simulink library "lib_TCML"  (R2015a)
settings: Solver=ode45  StartTime=0.0  StopTime=10.0  RelTol=1e-3
libraries: simulink x5
(part 3 of 7)

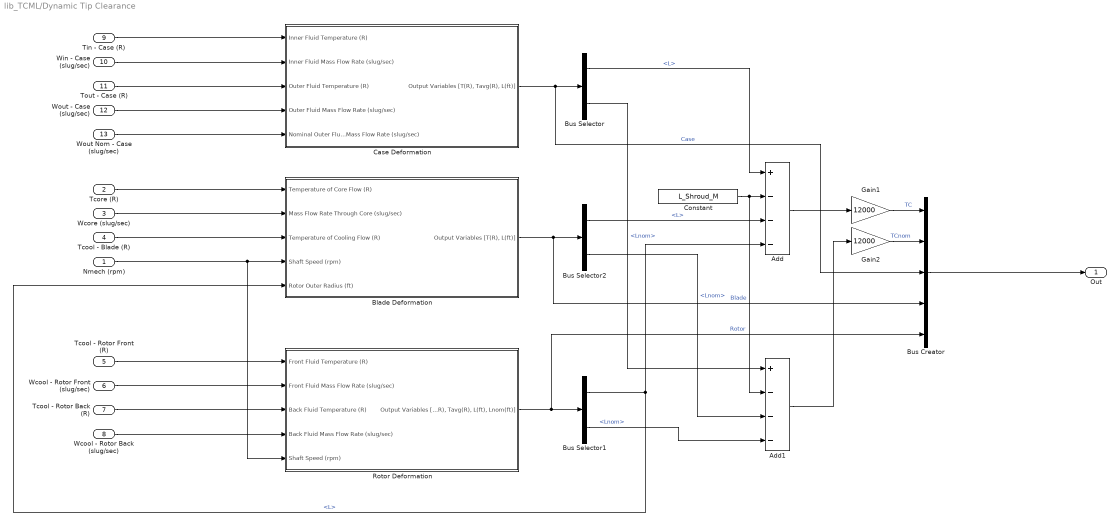
== system lib_TCML/Dynamic Tip Clearance ==
  Nmech (rpm) : Inport
  Tcore (R) : Inport  Port=2
  Wcore (slug/sec) : Inport  Port=3
  Tcool - Blade (R) : Inport  Port=4
  Tcool - Rotor Front (R) : Inport  Port=5
  Wcool - Rotor Front (slug/sec) : Inport  Port=6
  Tcool - Rotor Back (R) : Inport  Port=7
  Wcool - Rotor Back (slug/sec) : Inport  Port=8
  Tin - Case (R) : Inport  Port=9
  Win - Case (slug/sec) : Inport  Port=10
  Tout - Case (R) : Inport  Port=11
  Wout - Case (slug/sec) : Inport  Port=12
  Wout Nom - Case (slug/sec) : Inport  Port=13
  Add : Sum  Inputs=+---
  Add1 : Sum  Inputs=+---
  Blade Deformation : Subsystem
  Bus Creator : BusCreator  Inputs=5
  Bus Selector : BusSelector  OutputSignals=L,Lnom
  Bus Selector1 : BusSelector  OutputSignals=L,Lnom
  Bus Selector2 : BusSelector  OutputSignals=L,Lnom
  Case Deformation : Subsystem
  Constant : Constant  Value=L_Shroud_M
  Gain1 : Gain  Gain=12000
  Gain2 : Gain  Gain=12000
  Rotor Deformation : Subsystem
  Out : Outport
  wires:
  Add1/1 -> Gain2/1
  Bus Selector/2 -> Add1/1  "<Lnom>"
  Bus Selector2/2 -> Add1/3  "<Lnom>"
  Bus Selector1/2 -> Add1/4  "<Lnom>"
  Gain2/1 -> Bus Creator/2  "TCnom"
  Constant/1 -> Add/2, Add1/2
  Case Deformation/1("Output Variables [T(R), Tavg(R), L(ft)]") -> Bus Selector/1, Bus Creator/3  "Case"
  Wout - Case (slug/sec)/1 -> Case Deformation/4(Outer Fluid Mass Flow Rate (slug/sec))
  Tout - Case (R)/1 -> Case Deformation/3(Outer Fluid Temperature (R))
  Win - Case (slug/sec)/1 -> Case Deformation/2(Inner Fluid Mass Flow Rate (slug/sec))
  Tin - Case (R)/1 -> Case Deformation/1(Inner Fluid Temperature (R))
  Gain1/1 -> Bus Creator/1  "TC"
  Bus Selector/1 -> Add/1  "<L>"
  Bus Selector1/1 -> Add/4, Blade Deformation/5(Rotor Outer Radius (ft))  "<L>"
  Rotor Deformation/1("Output Variables [T(R), Tavg(R), L(ft), Lnom(ft)]") -> Bus Selector1/1, Bus Creator/5  "Rotor"
  Blade Deformation/1("Output Variables [T(R), L(ft)]") -> Bus Selector2/1, Bus Creator/4  "Blade"
  Bus Selector2/1 -> Add/3  "<L>"
  Add/1 -> Gain1/1
  Bus Creator/1 -> Out/1
  Tcore (R)/1 -> Blade Deformation/1(Temperature of Core Flow (R))
  Wcore (slug/sec)/1 -> Blade Deformation/2(Mass Flow Rate Through Core (slug/sec))
  Tcool - Blade (R)/1 -> Blade Deformation/3(Temperature of Cooling Flow (R))
  Nmech (rpm)/1 -> Blade Deformation/4(Shaft Speed (rpm)), Rotor Deformation/5(Shaft Speed (rpm))
  Tcool - Rotor Front (R)/1 -> Rotor Deformation/1(Front Fluid Temperature (R))
  Wcool - Rotor Front (slug/sec)/1 -> Rotor Deformation/2(Front Fluid Mass Flow Rate (slug/sec))
  Tcool - Rotor Back (R)/1 -> Rotor Deformation/3(Back Fluid Temperature (R))
  Wcool - Rotor Back (slug/sec)/1 -> Rotor Deformation/4(Back Fluid Mass Flow Rate (slug/sec))
  Wout Nom - Case (slug/sec)/1 -> Case Deformation/5(Nominal Outer Fluid Mass Flow Rate (slug/sec))

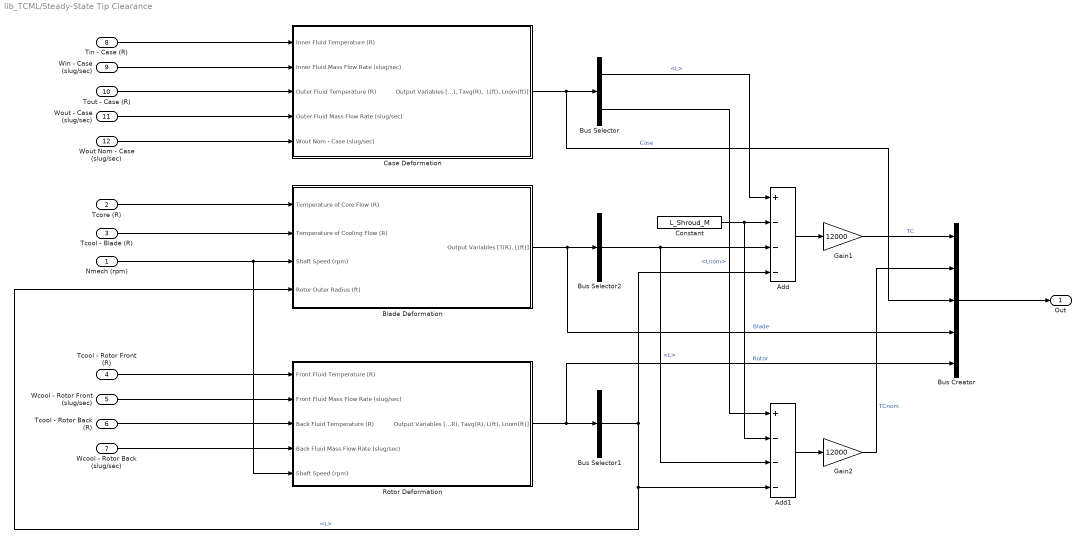
== system lib_TCML/Steady-State Tip Clearance ==
  Nmech (rpm) : Inport
  Tcore (R) : Inport  Port=2
  Tcool - Blade (R) : Inport  Port=3
  Tcool - Rotor Front (R) : Inport  Port=4
  Wcool - Rotor Front (slug/sec) : Inport  Port=5
  Tcool - Rotor Back (R) : Inport  Port=6
  Wcool - Rotor Back (slug/sec) : Inport  Port=7
  Tin - Case (R) : Inport  Port=8
  Win - Case (slug/sec) : Inport  Port=9
  Tout - Case (R) : Inport  Port=10
  Wout - Case (slug/sec) : Inport  Port=11
  Wout Nom - Case (slug/sec) : Inport  Port=12
  Add : Sum  Inputs=+---
  Add1 : Sum  Inputs=+---
  Blade Deformation : Subsystem
  Bus Creator : BusCreator  Inputs=5
  Bus Selector : BusSelector  OutputSignals=L,Lnom
  Bus Selector1 : BusSelector  OutputSignals=L
  Bus Selector2 : BusSelector  OutputSignals=L
  Case Deformation : Subsystem
  Constant : Constant  Value=L_Shroud_M
  Gain1 : Gain  Gain=12000
  Gain2 : Gain  Gain=12000
  Rotor Deformation : Subsystem
  Out : Outport
  wires:
  Tin - Case (R)/1 -> Case Deformation/1(Inner Fluid Temperature (R))
  Wcool - Rotor Back (slug/sec)/1 -> Rotor Deformation/4(Back Fluid Mass Flow Rate (slug/sec))
  Tcool - Rotor Back (R)/1 -> Rotor Deformation/3(Back Fluid Temperature (R))
  Wcool - Rotor Front (slug/sec)/1 -> Rotor Deformation/2(Front Fluid Mass Flow Rate (slug/sec))
  Tcool - Rotor Front (R)/1 -> Rotor Deformation/1(Front Fluid Temperature (R))
  Nmech (rpm)/1 -> Blade Deformation/3(Shaft Speed (rpm)), Rotor Deformation/5(Shaft Speed (rpm))
  Tcool - Blade (R)/1 -> Blade Deformation/2(Temperature of Cooling Flow (R))
  Wout - Case (slug/sec)/1 -> Case Deformation/4(Outer Fluid Mass Flow Rate (slug/sec))
  Tout - Case (R)/1 -> Case Deformation/3(Outer Fluid Temperature (R))
  Win - Case (slug/sec)/1 -> Case Deformation/2(Inner Fluid Mass Flow Rate (slug/sec))
  Tcore (R)/1 -> Blade Deformation/1(Temperature of Core Flow (R))
  Bus Creator/1 -> Out/1
  Case Deformation/1("Output Variables [T(R), Tavg(R),  L(ft), Lnom(ft)]") -> Bus Creator/3, Bus Selector/1  "Case"
  Add/1 -> Gain1/1
  Bus Selector2/1 -> Add/3, Add1/3  "<L>"
  Blade Deformation/1("Output Variables [T(R), L(ft)]") -> Bus Creator/4, Bus Selector2/1  "Blade"
  Rotor Deformation/1("Output Variables [T(R), Tavg(R), L(ft), Lnom(ft)]") -> Bus Creator/5, Bus Selector1/1  "Rotor"
  Bus Selector1/1 -> Add/4, Add1/4, Blade Deformation/4(Rotor Outer Radius (ft))  "<L>"
  Bus Selector/1 -> Add/1  "<L>"
  Gain1/1 -> Bus Creator/1  "TC"
  Wout Nom - Case (slug/sec)/1 -> Case Deformation/5(Wout Nom - Case (slug/sec))
  Add1/1 -> Gain2/1
  Bus Selector/2 -> Add1/1  "<Lnom>"
  Gain2/1 -> Bus Creator/2  "TCnom"
  Constant/1 -> Add1/2, Add/2

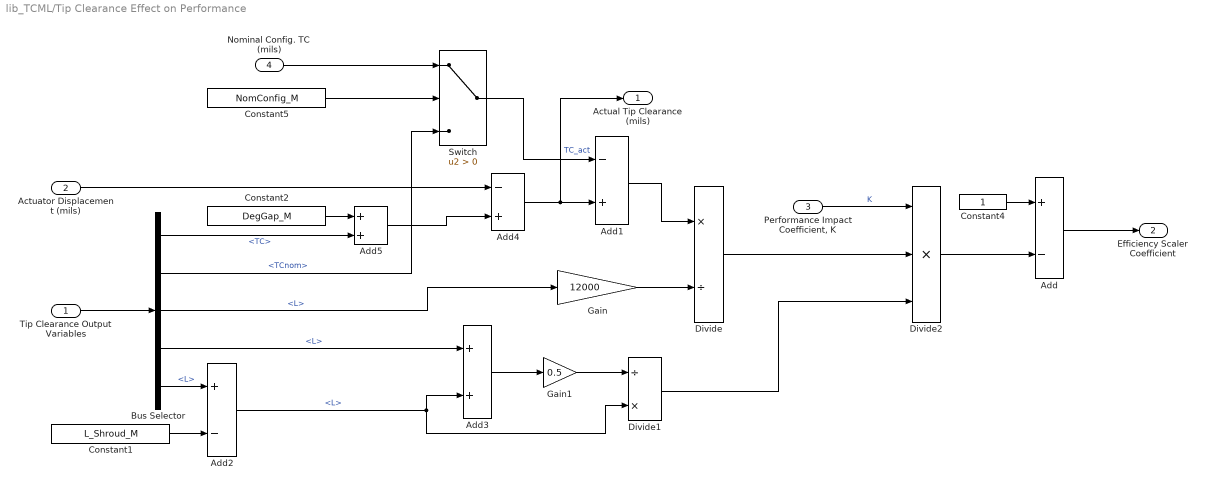
== system lib_TCML/Tip Clearance Effect on Performance ==
  Tip Clearance Output Variables : Inport
  Actuator Displacement (mils) : Inport  Port=2
  "Performance Impact Coefficient, K" : Inport  Port=3
  Nominal Config. TC (mils) : Inport  Port=4
  Add : Sum  Inputs=+-
  Add1 : Sum  Inputs=-+
  Add2 : Sum  Inputs=+-
  Add3 : Sum
  Add4 : Sum  Inputs=-+
  Add5 : Sum
  Bus Selector : BusSelector  OutputSignals=TC,TCnom,Blade.L,Rotor.L,Case.L
  Constant1 : Constant  Value=L_Shroud_M
  Constant2 : Constant  Value=DegGap_M
  Constant4 : Constant
  Constant5 : Constant  Value=NomConfig_M
  Divide : Product  Inputs=*/
  Divide1 : Product  Inputs=/*
  Divide2 : Product  Inputs=***
  Gain : Gain  Gain=12000
  Gain1 : Gain  Gain=0.5
  Switch : Switch  Criteria=u2 > Threshold
  Actual Tip Clearance (mils) : Outport
  Efficiency Scaler Coefficient : Outport  Port=2
  wires:
  Tip Clearance Output Variables/1 -> Bus Selector/1
  Constant4/1 -> Add/1
  Divide2/1 -> Add/2
  Divide/1 -> Divide2/2
  Add4/1 -> Actual Tip Clearance (mils)/1, Add1/2  "TC_act"
  Actuator Displacement (mils)/1 -> Add4/1
  Gain1/1 -> Divide1/1
  Add2/1 -> Add3/2, Divide1/2  "<L>"
  Bus Selector/3 -> Gain/1  "<L>"
  Add3/1 -> Gain1/1
  Bus Selector/1 -> Add5/2  "<TC>"
  "Performance Impact Coefficient, K"/1 -> Divide2/1  "K"
  Add1/1 -> Divide/1
  Bus Selector/4 -> Add3/1  "<L>"
  Divide1/1 -> Divide2/3
  Gain/1 -> Divide/2
  Add/1 -> Efficiency Scaler Coefficient/1
  Bus Selector/2 -> Switch/3  "<TCnom>"
  Constant1/1 -> Add2/2
  Bus Selector/5 -> Add2/1  "<L>"
  Add5/1 -> Add4/2
  Constant2/1 -> Add5/1
  Constant5/1 -> Switch/2
  Switch/1 -> Add1/1
  Nominal Config. TC (mils)/1 -> Switch/1

== system lib_TCML/Dynamic Tip Clearance/Blade Deformation ==
  Temperature of Core Flow (R) : Inport
  Mass Flow Rate Through Core (slug/sec) : Inport  Port=2
  Temperature of Cooling Flow (R) : Inport  Port=3
  Shaft Speed (rpm) : Inport  Port=4
  Rotor Outer Radius (ft) : Inport  Port=5
  Bus Creator : BusCreator
  Convective Heat Transfer Coefficient on Front Surface : Subsystem
  Deformation : Subsystem
  Deformation1 : Subsystem
  Lumped Mass Heat Transfer Model : Subsystem
  Rate Transition1 : RateTransition  X0=T0_Core_M  OutPortSampleTime=dt_Blade_M
  Rate Transition11 : RateTransition  X0=T0_Blade_M  OutPortSampleTime=dt_M
  Rate Transition2 : RateTransition  X0=T0_Core_M + eta_Blade_M*(Tcool0_Blade_M - T0_Core_M)  OutPortSampleTime=dt_M
  Rate Transition4 : RateTransition  X0=W0_Core_M  OutPortSampleTime=dt_Blade_M
  Temperature IC : Memory  X0=T0_Blade_M  InheritSampleTime=on
  Temperature of Core Flow (R) - Duplicate : InportShadow
  Thermal Properties : Subsystem
  "Output Variables [T(R), L(ft)]" : Outport
  wires:
  Deformation1/1(Blade Length) -> Bus Creator/4  "Lnom"
  Rate Transition2/1 -> Deformation1/1(Average Temperature)
  Lumped Mass Heat Transfer Model/2(Reference Temperature [Tref]) -> Rate Transition2/1
  Rotor Outer Radius (ft)/1 -> Deformation/3(Rotor Outer Radius), Deformation1/3(Rotor Outer Radius)
  Shaft Speed (rpm)/1 -> Deformation/2(Shaft Speed [N] (rpm)), Deformation1/2(Shaft Speed [N] (rpm))
  Temperature IC/1 -> Thermal Properties/1(Temperature [T])
  Mass Flow Rate Through Core (slug/sec)/1 -> Rate Transition4/1
  Temperature of Core Flow (R)/1 -> Rate Transition1/1
  Bus Creator/1 -> "Output Variables [T(R), L(ft)]"/1
  Deformation/1(Blade Length) -> Bus Creator/2  "L"
  Lumped Mass Heat Transfer Model/1(Blade Temperature [Tblade]) -> Rate Transition11/1, Temperature IC/1
  Thermal Properties/1(Heat Capacity [Cp]) -> Lumped Mass Heat Transfer Model/1(Heat Capacity of Blade)
  Convective Heat Transfer Coefficient on Front Surface/1(Convective Heat Transfer Coefficient [h]) -> Lumped Mass Heat Transfer Model/2(Convective Heat Transfer Coefficient)
  Temperature of Core Flow (R) - Duplicate/1 -> Lumped Mass Heat Transfer Model/3(Temperature of Core Flow [Tcore])
  Temperature of Cooling Flow (R)/1 -> Lumped Mass Heat Transfer Model/4(Temperature of Cooling Flow [Tcool])
  Rate Transition4/1 -> Convective Heat Transfer Coefficient on Front Surface/1(Mass Flow Rate [W])
  Rate Transition1/1 -> Convective Heat Transfer Coefficient on Front Surface/2(Fluid Temperature [T])
  Rate Transition11/1 -> Deformation/1(Average Temperature), Bus Creator/1  "T"
  Deformation/2(Unstrained Blade Length) -> Bus Creator/3  "Lu"

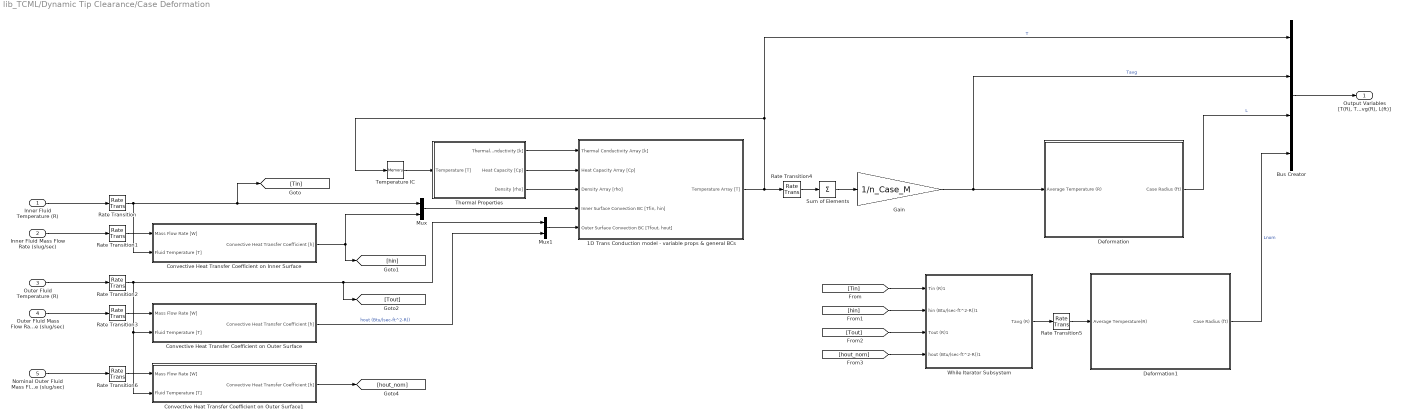
== system lib_TCML/Dynamic Tip Clearance/Case Deformation ==
  Inner Fluid Temperature (R) : Inport
  Inner Fluid Mass Flow Rate (slug/sec) : Inport  Port=2
  Outer Fluid Temperature (R) : Inport  Port=3
  Outer Fluid Mass Flow Rate (slug/sec) : Inport  Port=4
  Nominal Outer Fluid Mass Flow Rate (slug/sec) : Inport  Port=5
  1D Trans Conduction model - variable props & general BCs : Subsystem  mask(T-MATS: 1-D Trans Conduction Model - Variable Props + Generic BCs Block){x_M=x_Case_I, T0_M=T0_Case_M, dt_M=dt_Case_M, a_M=on, convin_M=on, radin_M=off, condin_M=off, convout_M=on, radout_M=off, condout_M=off, BN_M=double(gcb)}
      mask prompts: x_M "x_M - Discretized spatial domain (node locations) (nx1 array)"; T0_M "T0_M - Initial temperature array (nx1 array)"; dt_M "dt_M - Time step"; a_M "a_M - Shape (unchecked - planar, checked - cylindrical)"; convin_M "convin_M - Convection"; radin_M "radin_M - Radiation"; condin_M "condin_M - Conduction"; convout_M "convout_M - Convection"; radout_M "radout_M - Radiation"; condout_M "condout_M- Conduction"; BN_M "BN_M - Block name"
      mask help:
      | This function models the transient conduction of a 1-D structure which can either be of a planar or cylindrical geometry. This block solves the general 1-D heat equation using a finite difference method. It is able to handle variable thermal properties including density, heat capacity, and thermal conductivity. Abrupt transitions in material are also considered. It has the capability to address dynamic convection, conduction, and radiation boundary conditions. In addition, the discretized domain can be non-uniform but with the restriction that the boundary nodes should be half the thickness of their neighboring interior node (see the help menu).
      |
      | This block is able to accept inputs and parameters in a variety of units but it is important that the units be consistent. More details about this function, it's parameters, inputs, and outputs are provided in the help menu of this block.
      mask init:
      | % Setup Inports ----------------------------------------------------------%
      | 
      | % Inport Numbers
      | n = 4; %first BC inport number
      | 
      | % Inner Suface Convection Boundary Condition
      | if convin_M == 1
      |     if strcmp(get_param([BN_M '/Inner Surface Convection BC [Tfin, hin]'],'BlockType'),'Constant')
      |         MSK_ReplaceBlock_TMATS([BN_M '/Inner Surface Convection BC [Tfin, hin]'],'built-in/Inport');
      |     end
      |     set_param([BN_M '/Inner Surface Convection BC [Tfin, hin]'],'Port',num2str(n));
      |     n = n + 1;
      | elseif convin_M == 0
      |     if strcmp(get_param([BN_M '/Inner Surface Convection BC [Tfin, hin]'],'BlockType'),'Inport')
      |         MSK_ReplaceBlock_TMATS([BN_M '/Inner Surface Convection BC [Tfin, hin]'],'built-in/Constant');
      |         set_param([BN_M '/Inner Surface Convection BC [Tfin, hin]'],'Value','[0, 0]');
      |     end
      | end
      | 
      | % Inner Suface Radiation Boundary Condition
      | if radin_M == 1
      |     if strcmp(get_param([BN_M '/Inner Surface Radiation BC [Textin, uin]'],'BlockType'),'Constant')
      |         MSK_ReplaceBlock_TMATS([BN_M '/Inner Surface Radiation BC [Textin, uin]'],'built-in/Inport');
      |     end
      |     set_param([BN_M '/Inner Surface Radiation BC [Textin, uin]'],'Port',num2str(n));
      |     n = n + 1;
      | elseif radin_M == 0
      |     if strcmp(get_param([BN_M '/Inner Surface Radiation BC [Textin, uin]'],'BlockType'),'Inport')
      |         MSK_ReplaceBlock_TMATS([BN_M '/Inner Surface Radiation BC [Textin, uin]'],'built-in/Constant');
      |         set_param([BN_M '/Inner Surface Radiation BC [Textin, uin]'],'Value','[0, 0]');
      |     end
      | end
      | 
      | % Inner Suface Conduction Boundary Condition
      | if condin_M == 1
      |     if strcmp(get_param([BN_M '/Inner Surface Conduction BC [Tsin]'],'BlockType'),'Constant')
      |         MSK_ReplaceBlock_TMATS([BN_M '/Inner Surface Conduction BC [Tsin]'],'built-in/Inport');
      |     end
      |     set_param([BN_M '/Inner Surface Conduction BC [Tsin]'],'Port',num2str(n));
      |     n = n + 1;
      | elseif condin_M == 0
      |     if strcmp(get_param([BN_M '/Inner Surface Conduction BC [Tsin]'],'BlockType'),'Inport')
      |         MSK_ReplaceBlock_TMATS([BN_M '/Inner Surface Conduction BC [Tsin]'],'built-in/Constant');
      |         set_param([BN_M '/Inner Surface Conduction BC [Tsin]'],'Value','0');
      |     end
      | end
      | 
      | % Outer Suface Convection Boundary Condition
      | if convout_M == 1
      |     if strcmp(get_param([BN_M '/Outer Surface Convection BC [Tfout, hout]'],'BlockType'),'Constant')
      |         MSK_ReplaceBlock_TMATS([BN_M '/Outer Surface Convection BC [Tfout, hout]'],'built-in/Inport');
      |     end
      |     set_param([BN_M '/Outer Surface Convection BC [Tfout, hout]'],'Port',num2str(n));
      |     n = n + 1;
      | elseif convout_M == 0
      |     if strcmp(get_param([BN_M '/Outer Surface Convection BC [Tfout, hout]'],'BlockType'),'Inport')
      |         MSK_ReplaceBlock_TMATS([BN_M '/Outer Surface Convection BC [Tfout, hout]'],'built-in/Constant');
      |         set_param([BN_M '/Outer Surface Convection BC [Tfout, hout]'],'Value','[0, 0]');
      |     end
      | end
      | 
      | % Outer Suface Radiation Boundary Condition
      | if radout_M == 1
      |     if strcmp(get_param([BN_M '/Outer Surface Radiation BC [Textout, uout]'],'BlockType'),'Constant')
      |         MSK_ReplaceBlock_TMATS([BN_M '/Outer Surface Radiation BC [Textout, uout]'],'built-in/Inport');
      |     end
      |     set_param([BN_M '/Outer Surface Radiation BC [Textout, uout]'],'Port',num2str(n));
      |     n = n + 1;
      | elseif radout_M == 0
      |     if strcmp(get_param([BN_M '/Outer Surface Radiation BC [Textout, uout]'],'BlockType'),'Inport')
      |         MSK_ReplaceBlock_TMATS([BN_M '/Outer Surface Radiation BC [Textout, uout]'],'built-in/Constant');
      |         set_param([BN_M '/Outer Surface Radiation BC [Textout, uout]'],'Value','[0, 0]');
      |     end
      | end
      | 
      | % Outer Suface Conduction Boundary Condition
      | if condout_M == 1
      |     if strcmp(get_param([BN_M '/Outer Surface Conduction BC [Tsout]'],'BlockType'),'Constant')
      |         MSK_ReplaceBlock_TMATS([BN_M '/Outer Surface Conduction BC [Tsout]'],'built-in/Inport');
      |     end
      |     set_param([BN_M '/Outer Surface Conduction BC [Tsout]'],'Port',num2str(n));
      |     n = n + 1;
      | elseif condout_M == 0
      |     if strcmp(get_param([BN_M '/Outer Surface Conduction BC [Tsout]'],'BlockType'),'Inport')
      |         MSK_ReplaceBlock_TMATS([BN_M '/Outer Surface Conduction BC [Tsout]'],'built-in/Constant');
      |         set_param([BN_M '/Outer Surface Conduction BC [Tsout]'],'Value','0');
      |     end
      | end
      mask Help: web(which('HeatXfer_TMATS_1DTCondVarPropGenBC.html'),'-helpbrowser')
      mask DialogControl Container3 Prompt: General Parameters
      mask DialogControl Container4 Prompt: Active Inner Boundary Conditions
      mask DialogControl Container7 Prompt: Active Outer Boundary Conditions
  Bus Creator : BusCreator
  Convective Heat Transfer Coefficient on Inner Surface : Subsystem
  Convective Heat Transfer Coefficient on Outer Surface : Subsystem
  Convective Heat Transfer Coefficient on Outer Surface1 : Subsystem
  Deformation : Subsystem
  Deformation1 : Subsystem
  Gain : Gain  Gain=1/n_Case_M
  Mux : Mux  Inputs=2
  Mux1 : Mux  Inputs=2
  Rate Transition : RateTransition  X0=Tcool0_Case_In_M  OutPortSampleTime=dt_Case_M
  Rate Transition1 : RateTransition  X0=Wcool0_Case_In_M  OutPortSampleTime=dt_Case_M
  Rate Transition2 : RateTransition  X0=Tcool0_Case_Out_M  OutPortSampleTime=dt_Case_M
  Rate Transition3 : RateTransition  X0=Wcool0_Case_Out_M  OutPortSampleTime=dt_Case_M
  Rate Transition4 : RateTransition  X0=T0_Case_M  OutPortSampleTime=dt_M
  Rate Transition5 : RateTransition  X0=mean(T0_Case_M)  OutPortSampleTime=dt_M
  Rate Transition6 : RateTransition  X0=Wcool0_Case_Out_Nom_M  OutPortSampleTime=dt_Case_M
  Sum of Elements : Sum  Inputs=+
  Temperature IC : Memory  X0=T0_Case_M  InheritSampleTime=on
  Thermal Properties : Subsystem
  While Iterator Subsystem : Subsystem  TreatAsAtomicUnit=on
  "Output Variables [T(R), Tavg(R), L(ft)]" : Outport
  wires:
  Rate Transition5/1 -> Deformation1/1(Average Temperature(R))
  Deformation1/1(Case Radius (ft)) -> Bus Creator/4  "Lnom"
  While Iterator Subsystem/1(Tavg (R)) -> Rate Transition5/1
  [hout_nom] -> While Iterator Subsystem/4(hout (Btu/(sec-ft^2-R))1)
  [Tout] -> While Iterator Subsystem/3(Tout (R)1)
  [hin] -> While Iterator Subsystem/2(hin (Btu/(sec-ft^2-R))1)
  [Tin] -> While Iterator Subsystem/1(Tin (R)1)
  Convective Heat Transfer Coefficient on Inner Surface/1(Convective Heat Transfer Coefficient [h]) -> [hin], Mux/2
  Convective Heat Transfer Coefficient on Outer Surface/1(Convective Heat Transfer Coefficient [h]) -> Mux1/2  "hout (Btu/(sec-ft^2-R))"
  Rate Transition/1 -> Convective Heat Transfer Coefficient on Inner Surface/2(Fluid Temperature [T]), Mux/1, [Tin]
  Rate Transition2/1 -> Mux1/1, [Tout], Convective Heat Transfer Coefficient on Outer Surface1/2(Fluid Temperature [T]), Convective Heat Transfer Coefficient on Outer Surface/2(Fluid Temperature [T])
  1D Trans Conduction model - variable props & general BCs/1(Temperature Array [T]) -> Rate Transition4/1, Temperature IC/1, Bus Creator/1  "T"
  Rate Transition3/1 -> Convective Heat Transfer Coefficient on Outer Surface/1(Mass Flow Rate [W])
  Rate Transition1/1 -> Convective Heat Transfer Coefficient on Inner Surface/1(Mass Flow Rate [W])
  Deformation/1(Case Radius (ft)) -> Bus Creator/3  "L"
  Gain/1 -> Deformation/1(Average Temperature (R)), Bus Creator/2  "Tavg"
  Bus Creator/1 -> "Output Variables [T(R), Tavg(R), L(ft)]"/1
  Outer Fluid Temperature (R)/1 -> Rate Transition2/1
  Mux/1 -> 1D Trans Conduction model - variable props & general BCs/4("Inner Surface Convection BC [Tfin, hin]")
  Thermal Properties/1(Thermal Conductivity [k]) -> 1D Trans Conduction model - variable props & general BCs/1(Thermal Conductivity Array [k])
  Mux1/1 -> 1D Trans Conduction model - variable props & general BCs/5("Outer Surface Convection BC [Tfout, hout]")
  Inner Fluid Mass Flow Rate (slug/sec)/1 -> Rate Transition1/1
  Thermal Properties/3(Density [rho]) -> 1D Trans Conduction model - variable props & general BCs/3(Density Array [rho])
  Temperature IC/1 -> Thermal Properties/1(Temperature [T])
  Thermal Properties/2(Heat Capacity [Cp]) -> 1D Trans Conduction model - variable props & general BCs/2(Heat Capacity Array [Cp])
  Inner Fluid Temperature (R)/1 -> Rate Transition/1
  Outer Fluid Mass Flow Rate (slug/sec)/1 -> Rate Transition3/1
  Rate Transition4/1 -> Sum of Elements/1
  Sum of Elements/1 -> Gain/1
  Nominal Outer Fluid Mass Flow Rate (slug/sec)/1 -> Rate Transition6/1
  Rate Transition6/1 -> Convective Heat Transfer Coefficient on Outer Surface1/1(Mass Flow Rate [W])
  Convective Heat Transfer Coefficient on Outer Surface1/1(Convective Heat Transfer Coefficient [h]) -> [hout_nom]

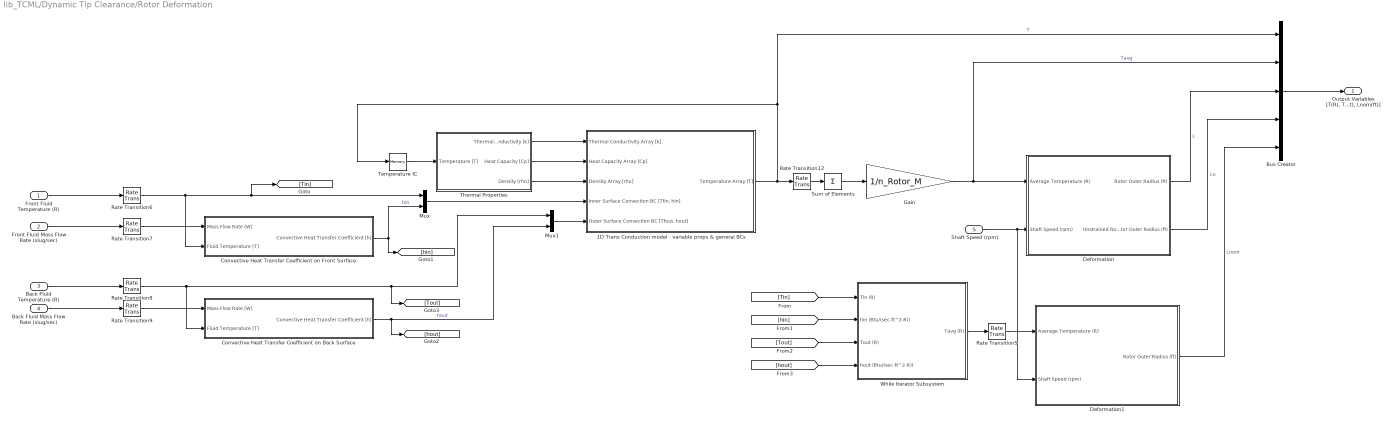
== system lib_TCML/Dynamic Tip Clearance/Rotor Deformation ==
  Front Fluid Temperature (R) : Inport
  Front Fluid Mass Flow Rate (slug/sec) : Inport  Port=2
  Back Fluid Temperature (R) : Inport  Port=3
  Back Fluid Mass Flow Rate (slug/sec) : Inport  Port=4
  Shaft Speed (rpm) : Inport  Port=5
  1D Trans Conduction model - variable props & general BCs : Subsystem  mask(T-MATS: 1-D Trans Conduction Model - Variable Props + Generic BCs Block){x_M=x_Rotor_I, T0_M=T0_Rotor_M, dt_M=dt_Rotor_M, a_M=off, convin_M=on, radin_M=off, condin_M=off, convout_M=on, radout_M=off, condout_M=off, BN_M=double(gcb)}
      mask prompts: x_M "x_M - Discretized spatial domain (node locations) (nx1 array)"; T0_M "T0_M - Initial temperature array (nx1 array)"; dt_M "dt_M - Time step"; a_M "a_M - Shape (unchecked - planar, checked - cylindrical)"; convin_M "convin_M - Convection"; radin_M "radin_M - Radiation"; condin_M "condin_M - Conduction"; convout_M "convout_M - Convection"; radout_M "radout_M - Radiation"; condout_M "condout_M- Conduction"; BN_M "BN_M - Block name"
      mask help:
      | This function models the transient conduction of a 1-D structure which can either be of a planar or cylindrical geometry. This block solves the general 1-D heat equation using a finite difference method. It is able to handle variable thermal properties including density, heat capacity, and thermal conductivity. Abrupt transitions in material are also considered. It has the capability to address dynamic convection, conduction, and radiation boundary conditions. In addition, the discretized domain can be non-uniform but with the restriction that the boundary nodes should be half the thickness of their neighboring interior node (see the help menu).
      |
      | This block is able to accept inputs and parameters in a variety of units but it is important that the units be consistent. More details about this function, it's parameters, inputs, and outputs are provided in the help menu of this block.
      mask init: same as lib_TCML/Dynamic Tip Clearance/Case Deformation/1D Trans Conduction model - variable props & general BCs
      mask Help: web(which('HeatXfer_TMATS_1DTCondVarPropGenBC.html'),'-helpbrowser')
      mask DialogControl Container3 Prompt: General Parameters
      mask DialogControl Container4 Prompt: Active Inner Boundary Conditions
      mask DialogControl Container7 Prompt: Active Outer Boundary Conditions
  Bus Creator : BusCreator  Inputs=5
  Convective Heat Transfer Coefficient on Back Surface : Subsystem
  Convective Heat Transfer Coefficient on Front Surface : Subsystem
  Deformation : Subsystem
  Deformation1 : Subsystem
  Gain : Gain  Gain=1/n_Rotor_M
  Mux : Mux  Inputs=2
  Mux1 : Mux  Inputs=2
  Rate Transition12 : RateTransition  X0=T0_Rotor_M  OutPortSampleTime=dt_M
  Rate Transition5 : RateTransition  X0=mean(T0_Rotor_M)  OutPortSampleTime=dt_M
  Rate Transition6 : RateTransition  X0=Tcool0_Rotor_Front_M  OutPortSampleTime=dt_Rotor_M
  Rate Transition7 : RateTransition  X0=Wcool0_Rotor_Front_M  OutPortSampleTime=dt_Rotor_M
  Rate Transition8 : RateTransition  X0=Tcool0_Rotor_Back_M  OutPortSampleTime=dt_Rotor_M
  Rate Transition9 : RateTransition  X0=Wcool0_Rotor_Back_M  OutPortSampleTime=dt_Rotor_M
  Sum of Elements : Sum  Inputs=+
  Temperature IC : Memory  X0=T0_Rotor_M  InheritSampleTime=on
  Thermal Properties : Subsystem
  While Iterator Subsystem : Subsystem  TreatAsAtomicUnit=on
  "Output Variables [T(R), Tavg(R), L(ft), Lnom(ft)]" : Outport
  wires:
  Deformation1/1(Rotor Outer Radius (ft)) -> Bus Creator/5  "Lnom"
  Rate Transition5/1 -> Deformation1/1(Average Temperature (R))
  While Iterator Subsystem/1(Tavg (R)) -> Rate Transition5/1
  [hout] -> While Iterator Subsystem/4(hout (Btu/(sec-ft^2-R)))
  [Tout] -> While Iterator Subsystem/3(Tout (R))
  [hin] -> While Iterator Subsystem/2(hin (Btu/(sec-ft^2-R)))
  [Tin] -> While Iterator Subsystem/1(Tin (R))
  Convective Heat Transfer Coefficient on Front Surface/1(Convective Heat Transfer Coefficient [h]) -> Mux/2, [hin]  "hin"
  Convective Heat Transfer Coefficient on Back Surface/1(Convective Heat Transfer Coefficient [h]) -> Mux1/2, [hout]  "hout"
  Shaft Speed (rpm)/1 -> Deformation/2(Shaft Speed (rpm)), Deformation1/2(Shaft Speed (rpm))
  Rate Transition8/1 -> [Tout], Mux1/1, Convective Heat Transfer Coefficient on Back Surface/2(Fluid Temperature [T])
  Rate Transition6/1 -> Mux/1, [Tin], Convective Heat Transfer Coefficient on Front Surface/2(Fluid Temperature [T])
  Mux1/1 -> 1D Trans Conduction model - variable props & general BCs/5("Outer Surface Convection BC [Tfout, hout]")
  Mux/1 -> 1D Trans Conduction model - variable props & general BCs/4("Inner Surface Convection BC [Tfin, hin]")
  Thermal Properties/3(Density [rho]) -> 1D Trans Conduction model - variable props & general BCs/3(Density Array [rho])
  Thermal Properties/1(Thermal Conductivity [k]) -> 1D Trans Conduction model - variable props & general BCs/1(Thermal Conductivity Array [k])
  Thermal Properties/2(Heat Capacity [Cp]) -> 1D Trans Conduction model - variable props & general BCs/2(Heat Capacity Array [Cp])
  Back Fluid Mass Flow Rate (slug/sec)/1 -> Rate Transition9/1
  1D Trans Conduction model - variable props & general BCs/1(Temperature Array [T]) -> Rate Transition12/1, Bus Creator/1, Temperature IC/1  "T"
  Front Fluid Mass Flow Rate (slug/sec)/1 -> Rate Transition7/1
  Temperature IC/1 -> Thermal Properties/1(Temperature [T])
  Gain/1 -> Bus Creator/2, Deformation/1(Average Temperature (R))  "Tavg"
  Deformation/1(Rotor Outer Radius (ft)) -> Bus Creator/3  "L"
  Front Fluid Temperature (R)/1 -> Rate Transition6/1
  Sum of Elements/1 -> Gain/1
  Back Fluid Temperature (R)/1 -> Rate Transition8/1
  Bus Creator/1 -> "Output Variables [T(R), Tavg(R), L(ft), Lnom(ft)]"/1
  Rate Transition7/1 -> Convective Heat Transfer Coefficient on Front Surface/1(Mass Flow Rate [W])
  Rate Transition9/1 -> Convective Heat Transfer Coefficient on Back Surface/1(Mass Flow Rate [W])
  Rate Transition12/1 -> Sum of Elements/1
  Deformation/2(Unstrained Rotor Outer Radius (ft)) -> Bus Creator/4  "Lu"

== system lib_TCML/Steady-State Tip Clearance/Blade Deformation ==
  Temperature of Core Flow (R) : Inport
  Temperature of Cooling Flow (R) : Inport  Port=2
  Shaft Speed (rpm) : Inport  Port=3
  Rotor Outer Radius (ft) : Inport  Port=4
  Bus Creator : BusCreator  Inputs=3
  Deformation : Subsystem
  Lumped Mass Heat Transfer Model : Subsystem
  "Output Variables [T(R), L(ft)]" : Outport
  wires:
  Temperature of Cooling Flow (R)/1 -> Lumped Mass Heat Transfer Model/2(Temperature of Cooling Flow [Tcool])
  Temperature of Core Flow (R)/1 -> Lumped Mass Heat Transfer Model/1(Temperature of Core Flow [Tcore])
  Shaft Speed (rpm)/1 -> Deformation/2(Shaft Speed [N] (rpm))
  Rotor Outer Radius (ft)/1 -> Deformation/3(Rotor Outer Radius)
  Deformation/1(Blade Length) -> Bus Creator/2  "L"
  Bus Creator/1 -> "Output Variables [T(R), L(ft)]"/1
  Lumped Mass Heat Transfer Model/1(Reference Temperature [Tref]) -> Deformation/1(Average Temperature), Bus Creator/1  "T"
  Deformation/2(Unstrained Blade Length) -> Bus Creator/3  "Lu"

== system lib_TCML/Steady-State Tip Clearance/Case Deformation ==
  Inner Fluid Temperature (R) : Inport
  Inner Fluid Mass Flow Rate (slug/sec) : Inport  Port=2
  Outer Fluid Temperature (R) : Inport  Port=3
  Outer Fluid Mass Flow Rate (slug/sec) : Inport  Port=4
  Wout Nom - Case (slug/sec) : Inport  Port=5
  Bus Creator : BusCreator
  Convective Heat Transfer Coefficient on Inner Surface : Subsystem
  Convective Heat Transfer Coefficient on Outer Surface : Subsystem
  Convective Heat Transfer Coefficient on Outer Surface1 : Subsystem
  Deformation : Subsystem
  Deformation1 : Subsystem
  Terminator : Terminator
  While Iterator Subsystem1 : Subsystem  TreatAsAtomicUnit=on
  While Iterator Subsystem2 : Subsystem  TreatAsAtomicUnit=on
  "Output Variables [T(R), Tavg(R),  L(ft), Lnom(ft)]" : Outport
  wires:
  While Iterator Subsystem1/2(Tavg (R)) -> Deformation/1(Average Temperature(R)), Bus Creator/2  "Tavg"
  Outer Fluid Temperature (R)/1 -> Convective Heat Transfer Coefficient on Outer Surface1/2(Fluid Temperature [T]), While Iterator Subsystem2/3(Tout (R)), Convective Heat Transfer Coefficient on Outer Surface/2(Fluid Temperature [T]), While Iterator Subsystem1/3(Tout (R))
  Inner Fluid Temperature (R)/1 -> While Iterator Subsystem1/1(Tin (R)), While Iterator Subsystem2/1(Tin (R)), Convective Heat Transfer Coefficient on Inner Surface/2(Fluid Temperature [T])
  While Iterator Subsystem1/1(T (R)) -> Bus Creator/1  "T"
  Outer Fluid Mass Flow Rate (slug/sec)/1 -> Convective Heat Transfer Coefficient on Outer Surface/1(Mass Flow Rate [W])
  Inner Fluid Mass Flow Rate (slug/sec)/1 -> Convective Heat Transfer Coefficient on Inner Surface/1(Mass Flow Rate [W])
  Bus Creator/1 -> "Output Variables [T(R), Tavg(R),  L(ft), Lnom(ft)]"/1
  Convective Heat Transfer Coefficient on Outer Surface/1(Convective Heat Transfer Coefficient [h]) -> While Iterator Subsystem1/4(hout (Btu/(sec-ft^2-R)))  "hout (Btu/(sec-ft^2-R))"
  Convective Heat Transfer Coefficient on Inner Surface/1(Convective Heat Transfer Coefficient [h]) -> While Iterator Subsystem2/2(hin (Btu/(sec-ft^2-R))), While Iterator Subsystem1/2(hin (Btu/(sec-ft^2-R)))  "hin (Btu/(sec-ft^2-R)"
  Deformation/1(Case Radius (ft)) -> Bus Creator/3  "L"
  Wout Nom - Case (slug/sec)/1 -> Convective Heat Transfer Coefficient on Outer Surface1/1(Mass Flow Rate [W])
  Convective Heat Transfer Coefficient on Outer Surface1/1(Convective Heat Transfer Coefficient [h]) -> While Iterator Subsystem2/4(hout (Btu/(sec-ft^2-R)))
  While Iterator Subsystem2/2(Tavg (R)) -> Deformation1/1(Average Temperature(R))
  While Iterator Subsystem2/1(T (R)) -> Terminator/1
  Deformation1/1(Case Radius (ft)) -> Bus Creator/4  "Lnom"

== system lib_TCML/Steady-State Tip Clearance/Rotor Deformation ==
  Front Fluid Temperature (R) : Inport
  Front Fluid Mass Flow Rate (slug/sec) : Inport  Port=2
  Back Fluid Temperature (R) : Inport  Port=3
  Back Fluid Mass Flow Rate (slug/sec) : Inport  Port=4
  Shaft Speed (rpm) : Inport  Port=5
  Bus Creator : BusCreator
  Convective Heat Transfer Coefficient on Back Surface : Subsystem
  Convective Heat Transfer Coefficient on Front Surface : Subsystem
  Deformation : Subsystem
  While Iterator Subsystem : Subsystem  TreatAsAtomicUnit=on
  "Output Variables [T(R), Tavg(R), L(ft), Lnom(ft)]" : Outport
  wires:
  While Iterator Subsystem/1(T (R)) -> Bus Creator/1  "T"
  Front Fluid Temperature (R)/1 -> While Iterator Subsystem/1(Tin (R)), Convective Heat Transfer Coefficient on Front Surface/2(Fluid Temperature [T])
  Back Fluid Mass Flow Rate (slug/sec)/1 -> Convective Heat Transfer Coefficient on Back Surface/1(Mass Flow Rate [W])
  Back Fluid Temperature (R)/1 -> While Iterator Subsystem/3(Tout (R)), Convective Heat Transfer Coefficient on Back Surface/2(Fluid Temperature [T])
  Front Fluid Mass Flow Rate (slug/sec)/1 -> Convective Heat Transfer Coefficient on Front Surface/1(Mass Flow Rate [W])
  Shaft Speed (rpm)/1 -> Deformation/2(Shaft Speed (rpm))
  Bus Creator/1 -> "Output Variables [T(R), Tavg(R), L(ft), Lnom(ft)]"/1
  Deformation/1(Rotor Outer Radius (ft)) -> Bus Creator/3  "L"
  Convective Heat Transfer Coefficient on Back Surface/1(Convective Heat Transfer Coefficient [h]) -> While Iterator Subsystem/4(hout (Btu/(sec-ft^2-R)))  "hout"
  Convective Heat Transfer Coefficient on Front Surface/1(Convective Heat Transfer Coefficient [h]) -> While Iterator Subsystem/2(hin (Btu/(sec-ft^2-R)))  "hin"
  While Iterator Subsystem/2(Tavg (R)) -> Deformation/1(Average Temperature (R)), Bus Creator/2  "Tavg"
  Deformation/2(Unstrained Rotor Outer Radius (ft)) -> Bus Creator/4  "Lu"

== system lib_TCML/Dynamic Tip Clearance/Blade Deformation/Convective Heat Transfer Coefficient on Front Surface ==
  Mass Flow Rate [W] : Inport
  Fluid Temperature [T] : Inport  Port=2
  2-D Lookup Table : Lookup_n-D  BreakpointsForDimension1=Wc_Blade_Data_M  BreakpointsForDimension2=Tc_Blade_Data_M  Table=h_Blade_Data_M  InternalRulePriority=Speed  RndMeth=Simplest  InputSameDT=on
  Constant : Constant  Value=0.8  SampleTime=dt_Blade_M
  Constant1 : Constant  Value=0.23  SampleTime=dt_Blade_M
  Convective Heat Transfer Coefficient : Constant  Value=h_Blade_M  SampleTime=dt_Blade_M
  Gain : Gain  Gain=hcoeff_Blade_M
  Gain1 : Gain  Gain=1/Wdes_Blade_M
  Gain2 : Gain  Gain=1/Tdes_Blade_M
  Math Function : Math  Operator=pow  SaturateOnIntegerOverflow=on
  Math Function1 : Math  Operator=pow  SaturateOnIntegerOverflow=on
  Multiport Switch : MultiPortSwitch
  Product : Product
  Which Convective Heat Transfer Coefficient Model? : Constant  Value=ConvHeatXCoeffMdl_Blade_I  SampleTime=dt_Blade_M
  Convective Heat Transfer Coefficient [h] : Outport
  wires:
  Product/1 -> Gain/1
  Math Function1/1 -> Product/2
  Math Function/1 -> Product/1
  Gain2/1 -> Math Function1/1, 2-D Lookup Table/1
  Fluid Temperature [T]/1 -> Gain2/1
  Constant1/1 -> Math Function1/2
  Gain1/1 -> Math Function/1, 2-D Lookup Table/2
  Convective Heat Transfer Coefficient/1 -> Multiport Switch/2
  Mass Flow Rate [W]/1 -> Gain1/1
  Gain/1 -> Multiport Switch/3
  Which Convective Heat Transfer Coefficient Model?/1 -> Multiport Switch/1
  Constant/1 -> Math Function/2
  2-D Lookup Table/1 -> Multiport Switch/4
  Multiport Switch/1 -> Convective Heat Transfer Coefficient [h]/1

== system lib_TCML/Dynamic Tip Clearance/Blade Deformation/Deformation ==
  Average Temperature : Inport
  Shaft Speed [N] (rpm) : Inport  Port=2
  Rotor Outer Radius : Inport  Port=3
  Deformation Due To Centrifugal Forces : Subsystem
  Deformation Due To Thermal Expansion : Subsystem
  Subtract : Sum
  Blade Length : Outport
  Unstrained Blade Length : Outport  Port=2
  wires:
  Average Temperature/1 -> Deformation Due To Thermal Expansion/1(Average Rotor Temperature), Deformation Due To Centrifugal Forces/2(Average Temperature)
  Subtract/1 -> Blade Length/1
  Shaft Speed [N] (rpm)/1 -> Deformation Due To Centrifugal Forces/1(Shaft Speed [N] (rpm))
  Deformation Due To Centrifugal Forces/1(Blade Length) -> Subtract/1
  Deformation Due To Thermal Expansion/1(Blade Length after Thermal Expansion) -> Unstrained Blade Length/1, Subtract/2, Deformation Due To Centrifugal Forces/3(Blade Length After Thermal Expansion)
  Rotor Outer Radius/1 -> Deformation Due To Centrifugal Forces/4(Rotor Outer Radius)

== system lib_TCML/Dynamic Tip Clearance/Blade Deformation/Deformation1 ==
  Average Temperature : Inport
  Shaft Speed [N] (rpm) : Inport  Port=2
  Rotor Outer Radius : Inport  Port=3
  Deformation Due To Centrifugal Forces : Subsystem
  Deformation Due To Thermal Expansion : Subsystem
  Subtract : Sum
  Blade Length : Outport
  wires:
  Rotor Outer Radius/1 -> Deformation Due To Centrifugal Forces/4(Rotor Outer Radius)
  Deformation Due To Thermal Expansion/1(Blade Length after Thermal Expansion) -> Deformation Due To Centrifugal Forces/3(Blade Length After Thermal Expansion), Subtract/2
  Deformation Due To Centrifugal Forces/1(Blade Length) -> Subtract/1
  Shaft Speed [N] (rpm)/1 -> Deformation Due To Centrifugal Forces/1(Shaft Speed [N] (rpm))
  Subtract/1 -> Blade Length/1
  Average Temperature/1 -> Deformation Due To Centrifugal Forces/2(Average Temperature), Deformation Due To Thermal Expansion/1(Average Blade Temperature)

== system lib_TCML/Dynamic Tip Clearance/Blade Deformation/Lumped Mass Heat Transfer Model ==
  Heat Capacity of Blade : Inport
  Convective Heat Transfer Coefficient : Inport  Port=2
  Temperature of Core Flow [Tcore] : Inport  Port=3
  Temperature of Cooling Flow [Tcool] : Inport  Port=4
  Add1 : Sum  Inputs=-+
  Add3 : Sum
  Add4 : Sum  Inputs=-+
  Constant2 : Constant  Value=A_Blade_M  SampleTime=dt_Blade_M
  Constant8 : Constant  Value=m_Blade_M  SampleTime=dt_Blade_M
  Divide : Product  Inputs=/**/*
  Gain : Gain  Gain=eta_Blade_M
  Integrator : Integrator  InitialCondition=T0_Blade_M
  Blade Temperature [Tblade] : Outport
  Reference Temperature [Tref] : Outport  Port=2
  wires:
  Divide/1 -> Integrator/1
  Add1/1 -> Gain/1
  Gain/1 -> Add3/2
  Add3/1 -> Add4/2, Reference Temperature [Tref]/1  "T ref"
  Constant8/1 -> Divide/4
  Constant2/1 -> Divide/2
  Add4/1 -> Divide/5  "deltaT"
  Temperature of Core Flow [Tcore]/1 -> Add1/1, Add3/1
  Temperature of Cooling Flow [Tcool]/1 -> Add1/2
  Convective Heat Transfer Coefficient/1 -> Divide/3
  Heat Capacity of Blade/1 -> Divide/1
  Integrator/1 -> Add4/1, Blade Temperature [Tblade]/1  "T"

== system lib_TCML/Dynamic Tip Clearance/Blade Deformation/Thermal Properties ==
  Temperature [T] : Inport
  Heat Capacity vs. Temperature : Lookup_n-D  NumberOfTableDimensions=1  BreakpointsForDimension1=TCp_Blade_Data_M  Table=Cp_Blade_Data_M  InternalRulePriority=Speed  RndMeth=Simplest  InputSameDT=on
  Is k of temperature dependent1 : Constant  Value=Cp_TempDependence_Blade_M  SampleTime=dt_Blade_M
  Switch1 : Switch  Criteria=u2 > Threshold
  Thermal Conductivity (Super Alloy)1 : Constant  Value=Cp_Blade_M  SampleTime=dt_Blade_M
  Heat Capacity [Cp] : Outport
  wires:
  Thermal Conductivity (Super Alloy)1/1 -> Switch1/3
  Heat Capacity vs. Temperature/1 -> Switch1/1
  Switch1/1 -> Heat Capacity [Cp]/1
  Is k of temperature dependent1/1 -> Switch1/2
  Temperature [T]/1 -> Heat Capacity vs. Temperature/1

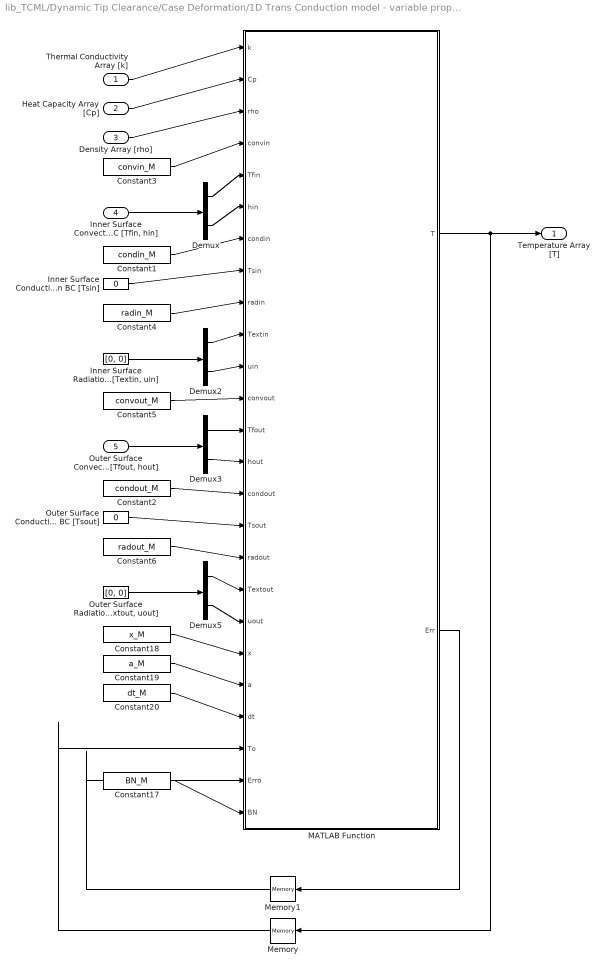
== system lib_TCML/Dynamic Tip Clearance/Case Deformation/1D Trans Conduction model - variable props & general BCs ==
  Thermal Conductivity Array [k] : Inport
  Heat Capacity Array [Cp] : Inport  Port=2
  Density Array [rho] : Inport  Port=3
  "Inner Surface Convection BC [Tfin, hin]" : Inport  Port=4
  "Outer Surface Convection BC [Tfout, hout]" : Inport  Port=5
  Constant1 : Constant  Value=condin_M
  Constant17 : Constant  Value=BN_M
  Constant18 : Constant  Value=x_M
  Constant19 : Constant  Value=a_M
  Constant2 : Constant  Value=condout_M
  Constant20 : Constant  Value=dt_M
  Constant3 : Constant  Value=convin_M
  Constant4 : Constant  Value=radin_M
  Constant5 : Constant  Value=convout_M
  Constant6 : Constant  Value=radout_M
  Demux{,2..3,5} (4 alike) : Demux  Outputs=[1 1]
  Inner Surface Conduction BC [Tsin] : Constant  Value=0
  "Inner Surface Radiation BC [Textin, uin]" : Constant  Value=[0, 0]
  MATLAB Function : MATLAB Function  TreatAsAtomicUnit=on  SystemSampleTime=dt_M
  Memory : Memory  X0=T0_M  InheritSampleTime=on
  Memory1 : Memory  X0=zeros(1,37)  InheritSampleTime=on
  Outer Surface Conduction BC [Tsout] : Constant  Value=0
  "Outer Surface Radiation BC [Textout, uout]" : Constant  Value=[0, 0]
  Temperature Array [T] : Outport
  wires:
  "Outer Surface Radiation BC [Textout, uout]"/1 -> Demux5/1
  Demux5/2 -> MATLAB Function/19(uout)
  Demux5/1 -> MATLAB Function/18(Textout)
  Outer Surface Conduction BC [Tsout]/1 -> MATLAB Function/16(Tsout)
  Demux3/2 -> MATLAB Function/14(hout)
  Demux3/1 -> MATLAB Function/13(Tfout)
  "Outer Surface Convection BC [Tfout, hout]"/1 -> Demux3/1
  Demux2/2 -> MATLAB Function/11(uin)
  Demux2/1 -> MATLAB Function/10(Textin)
  "Inner Surface Radiation BC [Textin, uin]"/1 -> Demux2/1
  Inner Surface Conduction BC [Tsin]/1 -> MATLAB Function/8(Tsin)
  Demux/2 -> MATLAB Function/6(hin)
  Demux/1 -> MATLAB Function/5(Tfin)
  "Inner Surface Convection BC [Tfin, hin]"/1 -> Demux/1
  Constant6/1 -> MATLAB Function/17(radout)
  Constant5/1 -> MATLAB Function/12(convout)
  Constant4/1 -> MATLAB Function/9(radin)
  Constant3/1 -> MATLAB Function/4(convin)
  Constant2/1 -> MATLAB Function/15(condout)
  Constant1/1 -> MATLAB Function/7(condin)
  MATLAB Function/2(Err) -> Memory1/1
  Memory/1 -> MATLAB Function/23(To)
  MATLAB Function/1(T) -> Temperature Array [T]/1, Memory/1
  Constant20/1 -> MATLAB Function/22(dt)
  Constant19/1 -> MATLAB Function/21(a)
  Constant18/1 -> MATLAB Function/20(x)
  Density Array [rho]/1 -> MATLAB Function/3(rho)
  Heat Capacity Array [Cp]/1 -> MATLAB Function/2(Cp)
  Thermal Conductivity Array [k]/1 -> MATLAB Function/1(k)
  Memory1/1 -> MATLAB Function/24(Erro)
  Constant17/1 -> MATLAB Function/25(BN)

== system lib_TCML/Dynamic Tip Clearance/Case Deformation/Convective Heat Transfer Coefficient on Inner Surface ==
  Mass Flow Rate [W] : Inport
  Fluid Temperature [T] : Inport  Port=2
  2-D Lookup Table : Lookup_n-D  BreakpointsForDimension1=Wc_Case_In_Data_M  BreakpointsForDimension2=Tc_Case_In_Data_M  Table=h_Case_In_Data_M  InternalRulePriority=Speed  RndMeth=Simplest  InputSameDT=on
  Constant : Constant  Value=0.8  SampleTime=dt_Case_M
  Constant1 : Constant  Value=0.23  SampleTime=dt_Case_M
  Convective Heat Transfer Coefficient : Constant  Value=h_Case_In_M  SampleTime=dt_Case_M
  Gain : Gain  Gain=hcoeff_Case_In_M
  Gain1 : Gain  Gain=1/Wdes_Case_In_M
  Gain2 : Gain  Gain=1/Tdes_Case_In_M
  Math Function : Math  Operator=pow  SaturateOnIntegerOverflow=on
  Math Function1 : Math  Operator=pow  SaturateOnIntegerOverflow=on
  Multiport Switch : MultiPortSwitch
  Product : Product
  Which Convective Heat Transfer Coefficient Model? : Constant  Value=ConvHeatXCoeffMdl_Case_In_I  SampleTime=dt_Case_M
  Convective Heat Transfer Coefficient [h] : Outport
  wires:
  Multiport Switch/1 -> Convective Heat Transfer Coefficient [h]/1
  2-D Lookup Table/1 -> Multiport Switch/4
  Constant/1 -> Math Function/2
  Which Convective Heat Transfer Coefficient Model?/1 -> Multiport Switch/1
  Gain/1 -> Multiport Switch/3
  Mass Flow Rate [W]/1 -> Gain1/1
  Convective Heat Transfer Coefficient/1 -> Multiport Switch/2
  Gain1/1 -> 2-D Lookup Table/2, Math Function/1
  Constant1/1 -> Math Function1/2
  Fluid Temperature [T]/1 -> Gain2/1
  Gain2/1 -> 2-D Lookup Table/1, Math Function1/1
  Math Function/1 -> Product/1
  Math Function1/1 -> Product/2
  Product/1 -> Gain/1

== system lib_TCML/Dynamic Tip Clearance/Case Deformation/Convective Heat Transfer Coefficient on Outer Surface ==
  Mass Flow Rate [W] : Inport
  Fluid Temperature [T] : Inport  Port=2
  2-D Lookup Table : Lookup_n-D  BreakpointsForDimension1=Wc_Case_Out_Data_M  BreakpointsForDimension2=Tc_Case_Out_Data_M  Table=h_Case_Out_Data_M  InternalRulePriority=Speed  RndMeth=Simplest  InputSameDT=on
  Constant : Constant  Value=0.8  SampleTime=dt_Case_M
  Constant1 : Constant  Value=0.23  SampleTime=dt_Case_M
  Convective Heat Transfer Coefficient : Constant  Value=h_Case_Out_M  SampleTime=dt_Case_M
  Gain : Gain  Gain=hcoeff_Case_Out_M
  Gain1 : Gain  Gain=1/Wdes_Case_Out_M
  Gain2 : Gain  Gain=1/Tdes_Case_Out_M
  Math Function : Math  Operator=pow  SaturateOnIntegerOverflow=on
  Math Function1 : Math  Operator=pow  SaturateOnIntegerOverflow=on
  Multiport Switch : MultiPortSwitch
  Product : Product
  Which Convective Heat Transfer Coefficient Model? : Constant  Value=ConvHeatXCoeffMdl_Case_Out_I  SampleTime=dt_Case_M
  Convective Heat Transfer Coefficient [h] : Outport
  wires:
  Product/1 -> Gain/1
  Math Function1/1 -> Product/2
  Math Function/1 -> Product/1
  Gain2/1 -> Math Function1/1, 2-D Lookup Table/1
  Fluid Temperature [T]/1 -> Gain2/1
  Constant1/1 -> Math Function1/2
  Gain1/1 -> Math Function/1, 2-D Lookup Table/2
  Convective Heat Transfer Coefficient/1 -> Multiport Switch/2
  Mass Flow Rate [W]/1 -> Gain1/1
  Gain/1 -> Multiport Switch/3
  Which Convective Heat Transfer Coefficient Model?/1 -> Multiport Switch/1
  Constant/1 -> Math Function/2
  2-D Lookup Table/1 -> Multiport Switch/4
  Multiport Switch/1 -> Convective Heat Transfer Coefficient [h]/1

== system lib_TCML/Dynamic Tip Clearance/Case Deformation/Convective Heat Transfer Coefficient on Outer Surface1 ==
  Mass Flow Rate [W] : Inport
  Fluid Temperature [T] : Inport  Port=2
  2-D Lookup Table : Lookup_n-D  BreakpointsForDimension1=Wc_Case_Out_Data_M  BreakpointsForDimension2=Tc_Case_Out_Data_M  Table=h_Case_Out_Data_M  InternalRulePriority=Speed  RndMeth=Simplest  InputSameDT=on
  Constant : Constant  Value=0.8  SampleTime=dt_Case_M
  Constant1 : Constant  Value=0.23  SampleTime=dt_Case_M
  Convective Heat Transfer Coefficient : Constant  Value=h_Case_Out_M  SampleTime=dt_Case_M
  Gain : Gain  Gain=hcoeff_Case_Out_M
  Gain1 : Gain  Gain=1/Wdes_Case_Out_M
  Gain2 : Gain  Gain=1/Tdes_Case_Out_M
  Math Function : Math  Operator=pow  SaturateOnIntegerOverflow=on
  Math Function1 : Math  Operator=pow  SaturateOnIntegerOverflow=on
  Multiport Switch : MultiPortSwitch
  Product : Product
  Which Convective Heat Transfer Coefficient Model? : Constant  Value=ConvHeatXCoeffMdl_Case_Out_I  SampleTime=dt_Case_M
  Convective Heat Transfer Coefficient [h] : Outport
  wires:
  Multiport Switch/1 -> Convective Heat Transfer Coefficient [h]/1
  2-D Lookup Table/1 -> Multiport Switch/4
  Constant/1 -> Math Function/2
  Which Convective Heat Transfer Coefficient Model?/1 -> Multiport Switch/1
  Gain/1 -> Multiport Switch/3
  Mass Flow Rate [W]/1 -> Gain1/1
  Convective Heat Transfer Coefficient/1 -> Multiport Switch/2
  Gain1/1 -> 2-D Lookup Table/2, Math Function/1
  Constant1/1 -> Math Function1/2
  Fluid Temperature [T]/1 -> Gain2/1
  Gain2/1 -> 2-D Lookup Table/1, Math Function1/1
  Math Function/1 -> Product/1
  Math Function1/1 -> Product/2
  Product/1 -> Gain/1

== system lib_TCML/Dynamic Tip Clearance/Case Deformation/Deformation ==
  Average Temperature (R) : Inport
  Memory : Memory  X0=mean(T0_Case_M)
  Memory3 : Memory  X0=Ri_Case_M
  Thermal Expansion 1D Elastic : Subsystem  mask(TSAT: Thermal Expansion Library Block){TempDependence_M=on, alpha_M=alpha_Case_M, T_data_M=Talpha_Case_Data_M, alpha_data_M=alpha_Case_Data_M, BN_M=double(gcb)}
      mask prompts: TempDependence_M "TempDependence_M - Temperature dependence of the thermal expansion coefficient (unchecked - constant, checked - temperature dependent)"; alpha_M "alpha_M - Constant thermal expansion coefficient"; T_data_M "T_data_M - Temperature array (nx1)"; alpha_data_M "alpha_data_M - Thermal expansion coefficient array (nx1)"; BN_M "Block Name"
      mask help:
      | This function calculates the length or radius of a structure that has expanded or contracted due to thermal expansion. The block accepts the previous/reference length (Lo), previous/reference temperature (To), and current temperature (Tf) as its inputs. The user has the option to specify a constant thermal expansion coefficient or to incorporate temperature dependence by providing data that correlates the thermal expansion coefficient with temperature.
      |
      | This block is capable of accepting various units but it is important that the units be consistent across all inputs and parameters. For details on this block, see the block help menu.
      mask init:
      | %set default parameters if they are not being used
      | if TempDependence_M == 0
      |     T_data_M = [0 5000];
      |     alpha_data_M = [10e-6 10e-6];
      | elseif TempDependence_M == 1
      |     alpha_M = 10e-6;
      | end
      mask Help: web(which('Deformation_TSAT_ThermExp1DElastic.html'),'-helpbrowser')
      mask Callback TempDependence_M:
      | MSK_SEC_Enables_TSAT('TempDependence_M',2,'dis')
      | MSK_SEC_Enables_TSAT('TempDependence_M',[3 4],'en')
  Case Radius (ft) : Outport
  wires:
  Thermal Expansion 1D Elastic/1(Current Length [L]) -> Memory3/1, Case Radius (ft)/1
  Average Temperature (R)/1 -> Memory/1, Thermal Expansion 1D Elastic/3(Current Temperature [Tf])
  Memory/1 -> Thermal Expansion 1D Elastic/2(Previous/Reference Temperature [To])
  Memory3/1 -> Thermal Expansion 1D Elastic/1(Previous/Reference Length [Lo])
